simulink model "FreeAcceleration"  (R2019b)
settings: Solver=ode8  StartTime=0.0  StopTime=2  FixedStep=0.0001  RelTol=1e-3  EnableMultiTasking=on
values from neighbouring files (symbols this model uses):
  B = inv([ ... (first row only)    [WECSConstants.m]
  H = 0.5    [WECSConstants.m]
  Xm = 2.042    [WECSConstants.m]
  Xr = Xlr+Xm    (= 2.0742)    [WECSConstants.m]
  Z = [ ... (first row only)    [WECSConstants.m]
libraries: powerlib_meascontrol x1
settings Model: Creator=Sony  LastModifiedBy=SONY
settings DataIOCC: LimitDataPoints=on  SaveFormat=Array  ReturnWorkspaceOutputs=off
settings OptimizationCC: LifeSpan=inf
settings DebuggingCC: UnderspecifiedInitializationDetection=Classic  MergeDetectMultiDrivingBlocksExec=none  SolverPrmCheckMsg=warning  StateNameClashWarn=warning  SFUnexpectedBacktrackingDiag=warning  SFNoUnconditionalDefaultTransitionDiag=warning  SFExecutionAtInitializationDiag=none  ArithmeticOperatorsInVariantConditions=warning
settings HardwareCC: ProdBitPerPointer=32  ProdBitPerSizeT=32  ProdBitPerPtrDiffT=32  ProdLargestAtomicFloat=None  ProdIntDivRoundTo=Undefined  ProdEndianess=Unspecified  ProdWordSize=32  ProdHWDeviceType=32-bit Generic
settings ModelReferenceCC: PropagateSignalLabelsOutOfModel=off
settings SFSimCC: SimUseLocalCustomCode=off  CustomCodeUndefinedFunction=UseInterfaceOnly
settings RTWCC: RTWUseLocalCustomCode=off
settings CodeAppCC: StateflowObjectComments=on
settings GRTTargetCC: TargetLangStandard=C89/C90 (ANSI)  GeneratePreprocessorConditionals=Disable all
settings ConfigComp: CovMetricSettings=dw  CovHtmlReporting=on  CovSaveCumulativeToWorkspaceVar=on  CovSaveSingleToWorkspaceVar=on  CovExternalEMLEnable=off

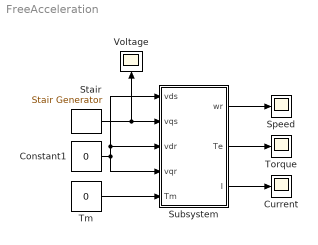
== system FreeAcceleration ==
  Constant1 : Constant  Value=0
  Current : Scope
  Speed : Scope
  Stair : powerlib_meascontrol/Pulse & Signal Generators/Stair Generator  t=[0, 0.5, 1]  e=[0, 1, 0]  Ts=0
      settings: SourceProductName=Simscape Electrical
  Subsystem : Subsystem
  Tm : Constant  Value=0
  Torque : Scope
  Voltage : Scope
  wires:
  Constant1/1 -> Subsystem/1(vds), Subsystem/3(vdr), Subsystem/4(vqr)
  Tm/1 -> Subsystem/5(Tm)
  Stair/1 -> Voltage/1, Subsystem/2(vqs)
  Subsystem/1(wr) -> Speed/1
  Subsystem/2(Te) -> Torque/1
  Subsystem/3(I) -> Current/1

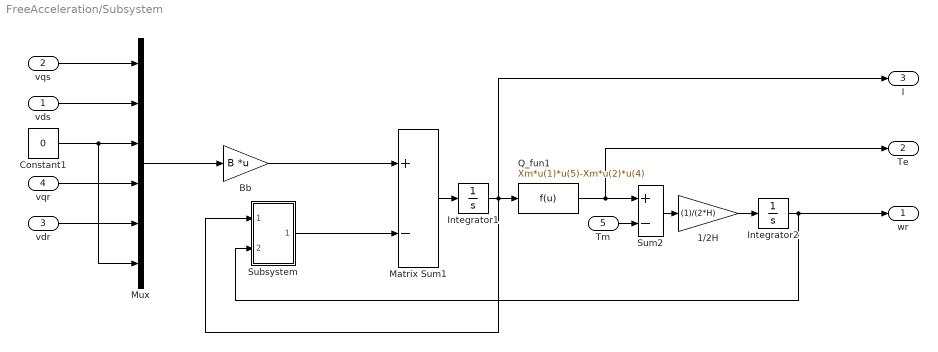
== system FreeAcceleration/Subsystem ==
  vds : Inport
  vqs : Inport  Port=2
  vdr : Inport  Port=3
  vqr : Inport  Port=4
  Tm : Inport  Port=5
  1/2H : Gain  Gain=(1)/(2*H)
  Bb : Gain  Gain=B  Multiplication=Matrix(K*u)
  Constant1 : Constant  Value=0
  Integrator1 : Integrator  InitialCondition=[0; 0; 0; 0; 0; 0]
  Integrator2 : Integrator
  Matrix Sum1 : Sum  Inputs=+-
  Mux : Mux  Inputs=6
  Q_fun1 : Fcn  Expr=Xm*u(1)*u(5)-Xm*u(2)*u(4)
  Subsystem : Subsystem
  Sum2 : Sum  Inputs=+-  SaturateOnIntegerOverflow=on  InputSameDT=on  OutDataTypeStr=Inherit: Same as first input
  wr : Outport
  Te : Outport  Port=2
  I : Outport  Port=3
  wires:
  Sum2/1 -> 1/2H/1
  vqs/1 -> Mux/1
  Matrix Sum1/1 -> Integrator1/1
  Constant1/1 -> Mux/6, Mux/3
  Tm/1 -> Sum2/2
  Q_fun1/1 -> Te/1, Sum2/1
  vds/1 -> Mux/2
  vdr/1 -> Mux/5
  Mux/1 -> Bb/1
  vqr/1 -> Mux/4
  1/2H/1 -> Integrator2/1
  Integrator1/1 -> Subsystem/1(In1), I/1, Q_fun1/1
  Bb/1 -> Matrix Sum1/1
  Integrator2/1 -> Subsystem/2(In2), wr/1
  Subsystem/1(Out1) -> Matrix Sum1/2

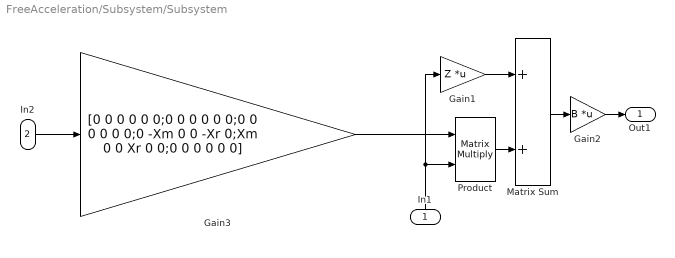
== system FreeAcceleration/Subsystem/Subsystem ==
  In1 : Inport
  In2 : Inport  Port=2
  Gain1 : Gain  Gain=Z  Multiplication=Matrix(K*u)
  Gain2 : Gain  Gain=B  Multiplication=Matrix(K*u)
  Gain3 : Gain  Gain=[0 0 0 0 0 0;0 0 0 0 0 0;0 0 0 0 0 0;0 -Xm 0 0 -Xr 0;Xm 0 0 Xr 0 0;0 0 0 0 0 0]
  Matrix Sum : Sum
  Product : Product  Multiplication=Matrix(*)
  Out1 : Outport
  wires:
  Gain2/1 -> Out1/1
  Product/1 -> Matrix Sum/2
  Matrix Sum/1 -> Gain2/1
  Gain3/1 -> Product/1
  Gain1/1 -> Matrix Sum/1
  In1/1 -> Product/2, Gain1/1
  In2/1 -> Gain3/1
